simulink model "Simulink_TF"  (R2020b)
settings: Solver=VariableStepAuto  StartTime=0.0  StopTime=4000  RelTol=1e-3
undefined symbols (not defined in the file): A, B, b, I, N, P, R, S, T
libraries: pid_lib x1
settings Model: Creator=jerem  LastModifiedBy=jerem

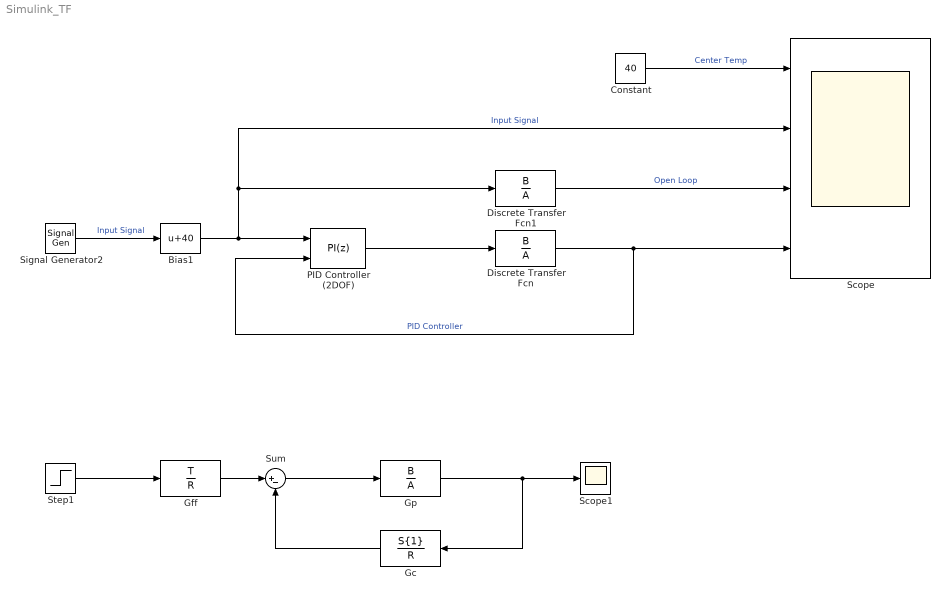
== system Simulink_TF ==
  Bias1 : Bias  Bias=40
  Constant : Constant  Value=40
  Discrete Transfer Fcn : DiscreteTransferFcn  Numerator=B  Denominator=A  SampleTime=0.4
  Discrete Transfer Fcn1 : DiscreteTransferFcn  Numerator=B  Denominator=A  SampleTime=0.4
  Gc : DiscreteTransferFcn  Numerator=S{1}  Denominator=R  SampleTime=0.4
  Gff : DiscreteTransferFcn  Numerator=T  Denominator=R  SampleTime=0.4
  Gp : DiscreteTransferFcn  Numerator=B  Denominator=A  SampleTime=0.4
  PID Controller (2DOF) : pid_lib/PID Controller (2DOF)  Controller=PI  Form=Parallel  TimeDomain=Discrete-time  UseExternalTs=off  SampleTime=0.4  IntegratorMethod=Forward Euler  FilterMethod=Forward Euler  ControllerParametersSource=internal  P=P  I=I  D=0  UseFilter=on  N=N  b=b  c=0  TunerSelectOption=Transfer Function Based (PID Tuner App)  InitialConditionSource=internal  InitialConditionForIntegrator=0  InitialConditionForFilter=0  DifferentiatorICPrevScaledInput=0  ExternalReset=none  TrackingMode=off  Kt=1  LimitOutput=off  SatLimitsSource=internal  UpperSaturationLimit=inf  LowerSaturationLimit=-inf  LinearizeAsGain=on  AntiWindupMode=none  Kb=1  POutMin=[]  POutMax=[]  IOutMin=[]  IOutMax=[]  DOutMin=[]  DOutMax=[]  NOutMin=[]  NOutMax=[]  bOutMin=[]  bOutMax=[]  cOutMin=[]  cOutMax=[]  SumOutMin=[]  SumOutMax=[]  SaturationOutMin=[]  SaturationOutMax=[]  PParamMin=[]  PParamMax=[]  IParamMin=[]  IParamMax=[]  DParamMin=[]  DParamMax=[]  NParamMin=[]  NParamMax=[]  bParamMin=[]  bParamMax=[]  cParamMin=[]  cParamMax=[]  KbParamMin=[]  KbParamMax=[]  KtParamMin=[]  KtParamMax=[]  KbOutMin=[]  KbOutMax=[]  KtOutMin=[]  KtOutMax=[]  IntegratorOutMin=[]  IntegratorOutMax=[]  FilterOutMin=[]  FilterOutMax=[]  SumI1OutMin=[]  SumI1OutMax=[]  SumI2OutMin=[]  SumI2OutMax=[]  SumI3OutMin=[]  SumI3OutMax=[]  SumI4OutMin=[]  SumI4OutMax=[]  SumDOutMin=[]  SumDOutMax=[]  Sum1OutMin=[]  Sum1OutMax=[]  Sum2OutMin=[]  Sum2OutMax=[]  Sum3OutMin=[]  Sum3OutMax=[]  DifferentiatorOutMin=[]  DifferentiatorOutMax=[]  FilterDiffOutCoefMin=[]  FilterDiffOutCoefMax=[]  ReciprocalOutMin=[]  ReciprocalOutMax=[]  SumDenOutMin=[]  SumDenOutMax=[]  SumNumOutMin=[]  SumNumOutMax=[]  DivideOutMin=[]  DivideOutMax=[]  UdiffTsProdOutMin=[]  UdiffTsProdOutMax=[]  NTsProdOutMin=[]  NTsProdOutMax=[]  UintegralTsProdOutMin=[]  UintegralTsProdOutMax=[]  UngainTsProdOutMin=[]  UngainTsProdOutMax=[]  IntegratorContinuousStateAttributes=''  IntegratorStateMustResolveToSignalObject=off  IntegratorRTWStateStorageClass=Auto  FilterContinuousStateAttributes=''  FilterStateMustResolveToSignalObject=off  FilterRTWStateStorageClass=Auto  ParallelPVariant=InternalParameters  IdealPVariant=Disabled  IVariant=InternalParameters  DVariant=Disabled  bVariant=InternalParameters  cVariant=Disabled  IntegratorVariant=Discrete  SatVariant=Disabled  AWVariant=Passthrough  PCopyVariant=Disabled  TRVariant=Disabled  FdbkBlocksVariant=Forward  IdealPFdbkVariant=Disabled  SatFdbkVariant=Disabled  DerivativeFilterVariant=Disabled  NVariant=Disabled  NCopyVariant=Disabled_SignalSpec  FilterICVariant=Disabled  IntegratorICVariant=InternalICs  ExternalResetVariant=Disabled  TRSumVariant=Passthrough  SumFdbkVariant=Disabled  SumVariant=Sum_PI  TsampFilterVariant=InternalTs  TsampNgainVariant=Passthrough  TsampIntegralVariant=Passthrough  ExternalSaturationOutDataTypeStr=Inherit: Same as second input
      settings: SourceProductBaseCode=SL
  Scope : Scope  NumInputPorts=4
  Scope1 : Scope
  Signal Generator2 : SignalGenerator  WaveForm=square  Amplitude=40  Frequency=1/1800
  Step1 : Step  SampleTime=0.4
  Sum : Sum  Inputs=|+-
  wires:
  Gp/1 -> Gc/1, Scope1/1
  Sum/1 -> Gp/1
  Discrete Transfer Fcn1/1 -> Scope/3  "Open Loop"
  Gff/1 -> Sum/1
  Step1/1 -> Gff/1
  Bias1/1 -> Scope/2, Discrete Transfer Fcn1/1, PID Controller (2DOF)/1  "Input Signal"
  PID Controller (2DOF)/1 -> Discrete Transfer Fcn/1
  Discrete Transfer Fcn/1 -> PID Controller (2DOF)/2, Scope/4  "PID Controller"
  Gc/1 -> Sum/2
  Signal Generator2/1 -> Bias1/1  "Input Signal"
  Constant/1 -> Scope/1  "Center Temp"
